simulink model "statelessWriter2_1"  (Simulink 9.1)
settings: Solver=VariableStepAuto  StartTime=0.0  StopTime=10.0  RelTol=1e-3
settings Model: SuppressorTable=22 serialization::archive 11 0 6 0 0 0 0 0  Creator=root  LastModifiedBy=BEAR
settings DataIOCC: SaveFormat=Dataset
settings OptimizationCC: LifeSpan=auto
settings DebuggingCC: UnderspecifiedInitializationDetection=Simplified  MergeDetectMultiDrivingBlocksExec=error  SFUnexpectedBacktrackingDiag=error  SFNoUnconditionalDefaultTransitionDiag=error  SFExecutionAtInitializationDiag=warning
settings HardwareCC: ProdBitPerPointer=64  ProdBitPerSizeT=64  ProdBitPerPtrDiffT=64  ProdLargestAtomicFloat=Float  ProdIntDivRoundTo=Zero  ProdEndianess=LittleEndian  ProdWordSize=64  ProdHWDeviceType=Intel->x86-64 (Windows64)
settings ModelReferenceCC: PropagateSignalLabelsOutOfModel=on
settings GRTTargetCC: TargetLangStandard=C99 (ISO)  CombineOutputUpdateFcns=on  GRTInterface=off
settings ConfigComp: CovMetricSettings=dwe  CovHtmlReporting=off  CovSaveCumulativeToWorkspaceVar=off  CovSaveSingleToWorkspaceVar=off  CovExternalEMLEnable=on

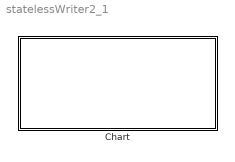
== system statelessWriter2_1 ==
  Chart : Stateflow chart  TreatAsAtomicUnit=on

== stateflow chart Chart ==
  settings: updateMethod=DISCRETE  sampleTime=2
  state idle
    en:heartbeat=0
    du:flag=1
  state pushing
    du:flag=0
  (default) -> idle : {i=3;cansend=1}
  pushing -> idle [order 1] : [i<=0]
  idle -> pushing [order 1] : [i>0]
  pushing -> pushing [order 2] : [cansend==1]{i=i-1}
  idle -> idle [order 2] : [after(3,sec)]{heartbeat=1}
  data: i local double; heartbeatPeriod constant double; flag local double; cansend local double; heartbeat local double; a local double
  events: event local FUNCTION_CALL_EVENT; event1 local FUNCTION_CALL_EVENT
